simulink library "PTOSim_Lib"  (R2021b)
settings: Solver=ode45  StartTime=0.0  StopTime=10.0  RelTol=1e-3  EnableMultiTasking=on
undefined symbols (not defined in the file or in its folder): DiscIntNeverNeededParam, PTOSimBlock, simu
libraries: $bdroot x3, simulink x2
(part 1 of 2)
settings Model: RequirementInfo="{}  %GIDa_42666abb_d6d9_408c_ae24_f6520282b61c"  Creator=sor  LastModifiedBy=jleonqu
settings SolverCC: AlgebraicLoopSolver=TrustRegion
settings DataIOCC: LimitDataPoints=on  SaveFormat=Array  ReturnWorkspaceOutputs=off
settings OptimizationCC: LifeSpan=inf
settings DebuggingCC: SolverPrmCheckMsg=warning  AllowSymbolicDim=off  SFUnexpectedBacktrackingDiag=warning  SFNoUnconditionalDefaultTransitionDiag=warning  SFExecutionAtInitializationDiag=none  SFMachineParentedDataDiag=warning  ArithmeticOperatorsInVariantConditions=warning
settings HardwareCC: ProdBitPerPointer=32  ProdBitPerSizeT=32  ProdBitPerPtrDiffT=32  ProdLargestAtomicFloat=None  ProdIntDivRoundTo=Undefined  ProdEndianess=Unspecified  ProdWordSize=32  ProdHWDeviceType=32-bit Generic
settings ModelReferenceCC: PropagateSignalLabelsOutOfModel=off
settings SFSimCC: SimUseLocalCustomCode=off  CustomCodeUndefinedFunction=UseInterfaceOnly
settings RTWCC: RTWUseLocalCustomCode=off
settings CodeAppCC: StateflowObjectComments=on
settings GRTTargetCC: TargetLangStandard=C89/C90 (ANSI)
settings ConfigComp: CovMetricSettings=dw  CovSaveCumulativeToWorkspaceVar=on  CovSaveSingleToWorkspaceVar=on  CovExternalEMLEnable=off  CovSFcnEnable=off

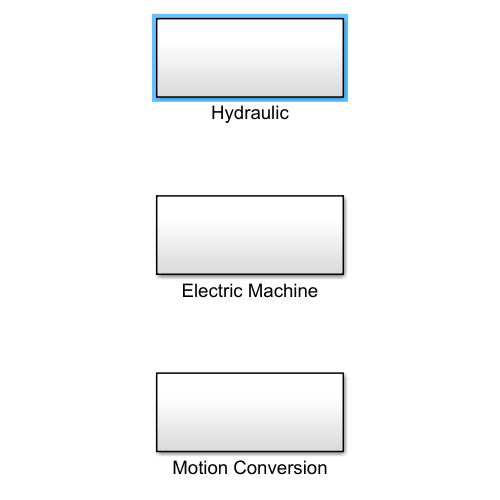
[thumbnail: Simulink's stored preview of the top-level diagram]
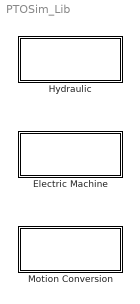
== system PTOSim_Lib ==
  Electric Machine : Subsystem  RequirementInfo="{}  %GIDa_5439fdb4_7c29_433c_8677_23bf92e18f11"
  Hydraulic : Subsystem  RequirementInfo={} %GIDa_f12a42eb_b9cb_4818_b573_b7dee4183a3b
  Motion Conversion : Subsystem

== system PTOSim_Lib/Electric Machine ==
  Electric Generator Equivalent Circuit : Subsystem  mask{PTOSimBlock=PTOSimBlock(1), InputFiletext=Use PTO-Sim input file to define Electric Machine parameters, Ra=0, La=0, Ke=0, bShaft=0, Jem=0}
      mask prompts: PTOSimBlock "Electric Machine Name"; Ra "Armature Resistance [ohm]"; La "Armature Inductance [H]"; Ke "Back-emf or Torque constant [V/(rad/s)]"; bShaft "Rotor Damping [N s/m]"; Jem "Rotor Inertia [kg m^2]"
      mask init:
      | if exist('PTOSimBlock','var')
      |     h=[gcb '/To Workspace'];
      |     responseName=['PTOSimBlock' num2str(PTOSimBlock.PTOSimBlockNum) '_out'];
      |     set_param(h,'VariableName',responseName);
      | end
      | clear h responseName
      | %HydraulicBlock.checkLoc('W');
      settings: PortSchema="{\"entries\":[{\"content\":{\"sides\":[{\"content\":{\"connectorIds\":[\"In1\"]},\"type\":\"ConnectorPlacement.EquallySpacedRectSide\",\"uuid\":\"38b15b7d-d952-45b6-9eb0-5d473736364e\"},{\"content\":{\"connectorIds\":[\"Out1\"],\"side\":\"RIGHT\"},\"type\":\"ConnectorPlacement.EquallySpacedRectSide\",\"uuid\":\"de64adb9-f2de-4dd5-b519-c63af884483d\"},{\"content\":{\"connectorIds\":[\"In2\"],\"side\":\"TOP\"},\"type\":\"ConnectorPlacement.EquallySpacedRectSide\",\"uuid\":\"eaa9506a-5e37-41b4-975c-a8d526700d36\"},{\"content\":{\"connectorIds\":[],\"side\":\"HIDDEN\"},\"type\":\"ConnectorPlacement.EquallySpacedRectSide\",\"uuid\":\"f8da1221-e5bc-4844-b966-beaaa1d6bf60\"}]},\"type\":\"ConnectorPlacement.EquallySpacedConnector\",\"uuid\":\"4da2b473-e94d-42dc-9143-64fbcbf5d9e1\"}],\"packageUris\":[\"http://schema.mathworks.com/mf0/Connector/R2020b\"],\"version\":\"1.0\"}"
      mask DialogControl ParameterGroupVar Prompt: Custom Parameters
      mask DialogControl EMParameters Prompt: Electric Machine Parameters
      mask Display: image('ElectricMotor.png'); % Use "Edit Image" on toolstrip to change.

== system PTOSim_Lib/Hydraulic ==
  Check Valve : Subsystem  mask{PTOSimBlock=PTOSimBlock(1), InputFileText=Use WEC-Sim input file to define Check Valve parameters, pMax=0, pMin=0, Amin=0, Amax=0, rho=0, cd=0, k1=0, k2=0}
      mask prompts: PTOSimBlock "Chack Valve Name"; pMax "Pressure difference at valve maximum opening [Pa]"; pMin "Pressure difference at valve minimum opening [Pa]"; Amin "Minimum valve area [m^2]"; Amax "Maximum valve area [m^2]"; rho "Fluid density [kg/m^3]"; cd "Discharge coefficient"; k1 "Valve coefficient k1 [m^2/N]"; k2 "Valve coefficient k2 [m^2/N]"
      mask init:
      | if exist('PTOSimBlock','var')
      |     h=[gcb '/To Workspace'];
      |     responseName=['PTOSimBlock' num2str(PTOSimBlock.PTOSimBlockNum) '_out'];
      |     set_param(h,'VariableName',responseName);
      | end
      | clear h responseName
      mask DialogControl ParameterGroupVar Prompt: Custom Parameters
      mask DialogControl CheckValveProperties Prompt: Check Valve Properties
      mask Display: image('CheckValve.png'); % Use "Edit Image" on toolstrip to change.
  Compressible Fluid Piston : Subsystem  mask{PTOSimBlock=PTOSimBlock(1), InputFileText=Use WEC-Sim input file to define the Conmpressible Fluid Piston parameters, Ap_A=0, Ap_B=0, PistonStroke=0, BulkModulus=0, xi_piston=0, pAi=0, pBi=0}
      mask prompts: PTOSimBlock "Piston Name"; Ap_A "Piston area A [m]"; Ap_B "Piston area B [m]"; PistonStroke "Piston stroke [m]"; BulkModulus "Fluid Bulk Modulus [Pa]"; xi_piston "Piston initial displacement from A [m]"; pAi "Port A Initial pressure [Pa]"; pBi "Port B Initial pressure [Pa]"
      mask help:
      | PTO-Sim Compressible Fluid Piston
      |
      | This block simualtes a hydraulic cylinder using a compressible fluid model. The block inputs are Response, QA and QB. Response is the signal output of the block Rotational PTO Actuation Force. QA and QB are the flow rate for port A and port B of the cylinder. The outputs of the block are ForcePTO, PA, and PB.
      mask init: same as PTOSim_Lib/Electric Machine/Electric Generator Equivalent Circuit
      settings: PortSchema="{\"entries\":[{\"content\":{\"sides\":[{\"content\":{\"connectorIds\":[\"In1\",\"In2\"]},\"type\":\"ConnectorPlacement.EquallySpacedRectSide\",\"uuid\":\"572dbc7c-8f4c-46fc-9000-663c89355fbd\"},{\"content\":{\"connectorIds\":[\"Out1\",\"Out2\",\"Out3\"],\"side\":\"RIGHT\"},\"type\":\"ConnectorPlacement.EquallySpacedRectSide\",\"uuid\":\"3b7821ce-a540-4de1-8f34-0d55375c774c\"},{\"content\":{\"connectorIds\":[\"In3\"],\"side\":\"TOP\"},\"type\":\"ConnectorPlacement.EquallySpacedRectSide\",\"uuid\":\"b6f5c275-868d-447d-b609-cdda14e9f222\"},{\"content\":{\"connectorIds\":[],\"side\":\"HIDDEN\"},\"type\":\"ConnectorPlacement.EquallySpacedRectSide\",\"uuid\":\"5b34aa5d-01fb-4d75-9f22-3e4ce64ee132\"}]},\"type\":\"ConnectorPlacement.EquallySpacedConnector\",\"uuid\":\"5b16a2f7-6624-4a26-89bf-8d87cef610e1\"}],\"packageUris\":[\"http://schema.mathworks.com/mf0/Connector/R2020b\"],\"version\":\"1.0\"}"
      mask Help:
      | This block simualtes a hydraulic cylinder using a compressible fluid model. The block inputs are Response and HydraulicInput. Response is the signal output of the block Rotational PTO Actuation Force. HydraulicInput is a two signal vector with the information of the flow rate for port A and port B of the cylinder. The output of the block is PistonOutput, which is a three signal vector with PressureA, PressureB, and ForcePTO.
      | 
      | The outputs are calculated using the model presented in the following link: http://wec-sim.github.io/WEC-Sim/master/user/advanced_features.html#pto-sim
      mask DialogControl ParameterGroupVar Prompt: Custom Parameters
      mask DialogControl PistonProperties Prompt: Piston Properties
      mask DialogControl InitialConditions Prompt: Initial Conditions
      mask Display: image('DoubleActingPiston.png'); % Use "Edit Image" on toolstrip to change.
  Gas-Charged Hydraulic Accumulator : Subsystem  mask{PTOSimBlock=PTOSimBlock(1), InputFileText=Use WEC-Sim input file to define Hydraulic Accumulator parameters, VI0=0, VIeq=0, pIprecharge=0}
      mask prompts: PTOSimBlock "Accumulator Name"; VI0 "Total Volume [m^3]"; VIeq "Initial Volume [m^3]"; pIprecharge "Precharge [Pa]"
      mask init: same as PTOSim_Lib/Electric Machine/Electric Generator Equivalent Circuit
      mask DialogControl ParameterGroupVar Prompt: Custom Parameters
      mask DialogControl AccProperties Prompt: Accumulator Properties
      mask Display: image('GasAccumulator.png'); % Use "Edit Image" on toolstrip to change.
  Hydraulic Motor : Subsystem  Variant=on  AllowZeroVariantControls=on  mask{PTOSimBlock=PTOSimBlock(1), InputFileText=Use WEC-Sim input file to define PTO parameters, Displacement=0, effModelVar=Analytical, EffTableDeltaP=0, EffTableShaftSpeed=0, EffTableMechEff=0, EffTableVolEff=0, wNominal=0, deltaPNominal=0, VisNominal=0, DensityNominal=0, EffVolNom=0, TorqueNoLoad=0, TorqueVsPressure=0, rho=0, Viscosity=0}
      mask prompts: PTOSimBlock "Hydraulic Motor Name"; Displacement "Displacement [cc/rev]"; effModelVar "Efficiency Model"; EffTableDeltaP "Pressure data [Pa]"; EffTableShaftSpeed "Shaft speed data [rpm]"; EffTableMechEff "Mechanical Efficiency"; EffTableVolEff "Volumetric Efficiency"; wNominal "Nominal shaft speed [rpm]"; deltaPNominal "Nominal pressure [Pa]"; VisNominal "Nominal viscosity [m^2/s]"; DensityNominal "Nominal density [kg/m^3]"; EffVolNom "Nominal volumetric efficiency"; TorqueNoLoad "No load torque [Nm]"; TorqueVsPressure "Friction torque vs pressure coefficient [Nm/Pa]"; rho "Fluid density [kg/m^3]"; Viscosity "Fluid viscosity [m^2/s]"
      mask init:
      | if exist('PTOSimBlock','var')
      |     %%
      |     % Analytical efficiency
      |     %%
      |     h = [gcb '/AnalyticalEfficiencyModel'];
      |     responseName = ['sv_b' num2str(PTOSimBlock.PTOSimBlockNum) '_AnalyticalEfficiency'];
      |     set_param(h,'VariantControl',responseName);
      |     %%
      |     % Tabulated Efficiency
      |     %%
      |     h = [gcb '/TabulatedEfficiency'];
      |     responseName = ['sv_b' num2str(PTOSimBlock.PTOSimBlockNum) '_TabulatedEfficiency'];
      |     set_param(h,'VariantControl',responseName);
      |     %%
      |     % Set zero active variant controls to prevent label issue (works 2017b+)
      |     %%
      |     set_param(gcb,'AllowZeroVariantControls','on');
      |     %%
      |     h=[gcb '/TabulatedEfficiency/To Workspace'];
      |     responseName=['PTOSimBlock' num2str(PTOSimBlock.PTOSimBlockNum) '_out'];
      |     set_param(h,'VariableName',responseName);
      |     %%
      |     h=[gcb '/AnalyticalEfficiencyModel/To Workspace'];
      |     responseName=['PTOSimBlock' num2str(PTOSimBlock.PTOSimBlockNum) '_out'];
      |     set_param(h,'VariableName',responseName);
      | end
      | clear h responseName
      mask TypeOptions effModelVar: Analytical | Tabulated
      mask Callback effModelVar: ptoSimClassCallback(gcbh)
      mask DialogControl ParameterGroupVar Prompt: Custom Parameters
      mask DialogControl HMProperties Prompt: Hydraulic Motor Properties
      mask Display: image('VariableDisplacementHydraulicMotor.png'); % Use "Edit Image" on toolstrip to change.
  Rectifying Check Valve : Subsystem  mask{PTOSimBlock=PTOSimBlock(1), InputFileText=Use PTO-Sim input file to define PTO parameters, Cd=0, Amax=0, Amin=0, pMin=0, pMax=0, rho=0, k1=0, k2=0}
      mask prompts: PTOSimBlock "Rectifying Valve Name"; Cd "Discharge coefficient"; Amax "Maximum opening area"; Amin "Minimum opening Area"; pMin "Cracking pressure"; pMax "Pressure at maximum opening"; rho "Fluid density"; k1 "Valve Coefficient k1"; k2 "Valve Coefficient k2"
      mask init: same as PTOSim_Lib/Electric Machine/Electric Generator Equivalent Circuit
      mask DialogControl ParameterGroupVar Prompt: Custom Parameters
      mask DialogControl CheckValveProperties Prompt: Check valve properties
      mask Display: image('RectifyingCheckValve.png'); % Use "Edit Image" on toolstrip to change.

== system PTOSim_Lib/Motion Conversion ==
  Rotary to Linear Adjustable Rod : Subsystem  mask{PTOSimBlock=PTOSimBlock(1), InputFiletext=Use WEC-Sim input file to define Adjustable Rod parameters, crank=0, offset=0, rodInit=0}
      mask prompts: PTOSimBlock "Adjustable Rod Name"; crank "Crank [m]"; offset "Offset [m]"; rodInit "Rod initial position [m]"
      mask init: same as PTOSim_Lib/Hydraulic/Check Valve
      mask DialogControl ParameterGroupVar Prompt: Custom Parameters
      mask DialogControl AdjRodParameters Prompt: Adjustable Rod Properties
  Rotary to Linear Crank : Subsystem  mask{PTOSimBlock=PTOSimBlock(1), InputFiletext=Use WEC-Sim input file to define Linear Crank parameters, crank=0, offset=0, rodLength=0}
      mask prompts: PTOSimBlock "Linear Crank Name"; crank "Crank [m]"; offset "Offset [m]"; rodLength "Rod length [m]"
      mask init: same as PTOSim_Lib/Hydraulic/Check Valve
      mask DialogControl ParameterGroupVar Prompt: Custom Parameters
      mask DialogControl LinCrankParameters Prompt: Linear Crank Parameters

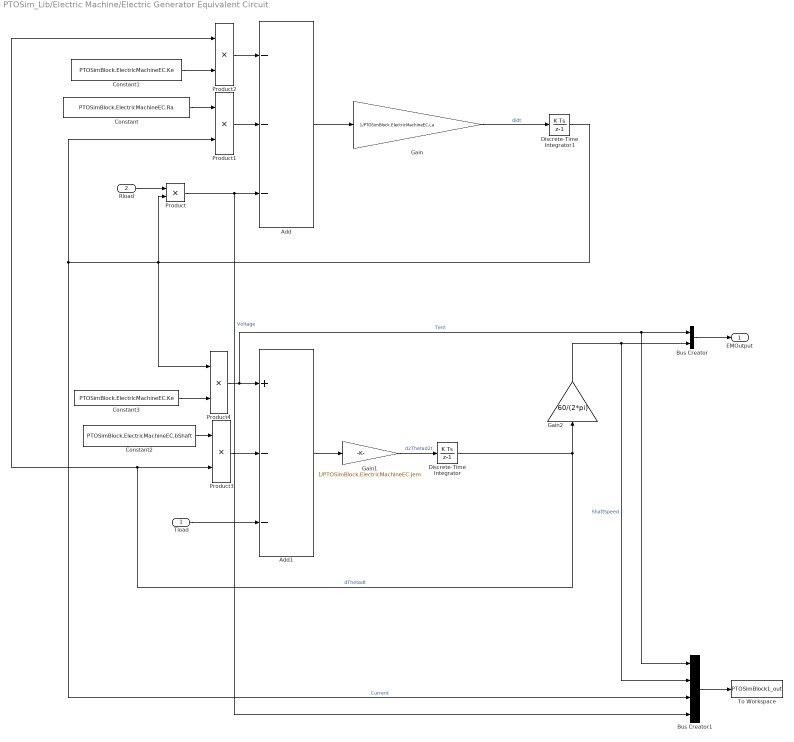
== system PTOSim_Lib/Electric Machine/Electric Generator Equivalent Circuit ==
  Tload : Inport
  Rload : Inport  Port=2
  Add : Sum  Inputs=---
  Add1 : Sum  Inputs=+--
  Bus Creator : BusCreator  Inputs=2
  Bus Creator1 : BusCreator  Inputs=4
  Constant : Constant  Value=PTOSimBlock.ElectricMachineEC.Ra
  Constant1 : Constant  Value=PTOSimBlock.ElectricMachineEC.Ke
  Constant2 : Constant  Value=PTOSimBlock.ElectricMachineEC.bShaft
  Constant3 : Constant  Value=PTOSimBlock.ElectricMachineEC.Ke
  Discrete-Time Integrator : DiscreteIntegrator  SampleTime=-1  ICPrevOutput=DiscIntNeverNeededParam  ICPrevScaledInput=DiscIntNeverNeededParam
  Discrete-Time Integrator1 : DiscreteIntegrator  SampleTime=-1  ICPrevOutput=DiscIntNeverNeededParam  ICPrevScaledInput=DiscIntNeverNeededParam
  Gain : Gain  Gain=1/PTOSimBlock.ElectricMachineEC.La
  Gain1 : Gain  Gain=1/PTOSimBlock.ElectricMachineEC.Jem
  Gain2 : Gain  Gain=60/(2*pi)
  Product{,1..4} (5 alike) : Product
  To Workspace : ToWorkspace  VariableName=PTOSimBlock1_out  SaveFormat=Structure With Time  SampleTime=simu.dtOut
  EMOutput : Outport
  wires:
  Add/1 -> Gain/1
  Gain/1 -> Discrete-Time Integrator1/1  "didt"
  Rload/1 -> Product/1
  Discrete-Time Integrator1/1 -> Product4/1, Product/2, Bus Creator1/3, Product1/2  "Current"
  Product/1 -> Bus Creator1/4, Add/3  "Voltage"
  Product1/1 -> Add/2
  Constant/1 -> Product1/1
  Product2/1 -> Add/1
  Constant1/1 -> Product2/2
  Tload/1 -> Add1/3
  Add1/1 -> Gain1/1
  Gain1/1 -> Discrete-Time Integrator/1  "d2Thetad2t"
  Product3/1 -> Add1/2
  Constant2/1 -> Product3/1
  Discrete-Time Integrator/1 -> Product2/1, Product3/2, Gain2/1  "dThetadt"
  Product4/1 -> Bus Creator1/1, Bus Creator/1, Add1/1  "Tem"
  Constant3/1 -> Product4/2
  Bus Creator/1 -> EMOutput/1
  Gain2/1 -> Bus Creator1/2, Bus Creator/2  "ShaftSpeed"
  Bus Creator1/1 -> To Workspace/1

== system PTOSim_Lib/Hydraulic/Check Valve ==
  DeltaP : Inport
  Bus Creator : BusCreator  Inputs=2
  Constant : Constant  Value=PTOSimBlock.CheckValve.rho
  Divide : Product  Inputs=/*
  Gain : Gain  Gain=PTOSimBlock.CheckValve.k1
  Gain1 : Gain  Gain=2
  Gain2 : Gain  Gain=PTOSimBlock.CheckValve.Cd
  Product : Product
  Product1 : Product
  Sqrt : Sqrt  SaturateOnIntegerOverflow=on
  Subsystem : Subsystem
  To Workspace : ToWorkspace  VariableName=PTOSimBlock1_out  SaveFormat=Structure With Time  SampleTime=-1
  Trigonometric Function : Trigonometry  Operator=tanh
  Qcv : Outport
  wires:
  Product1/1 -> Bus Creator/1, Qcv/1  "FlowCheckValve"
  DeltaP/1 -> Bus Creator/2, Subsystem/1(DeltaP), Gain/1, Gain1/1  "DeltaPCheckValve"
  Subsystem/1(Av) -> Product1/2
  Gain/1 -> Trigonometric Function/1
  Trigonometric Function/1 -> Product/1
  Gain1/1 -> Product/2
  Sqrt/1 -> Gain2/1
  Divide/1 -> Sqrt/1
  Gain2/1 -> Product1/1
  Constant/1 -> Divide/1
  Product/1 -> Divide/2
  Bus Creator/1 -> To Workspace/1

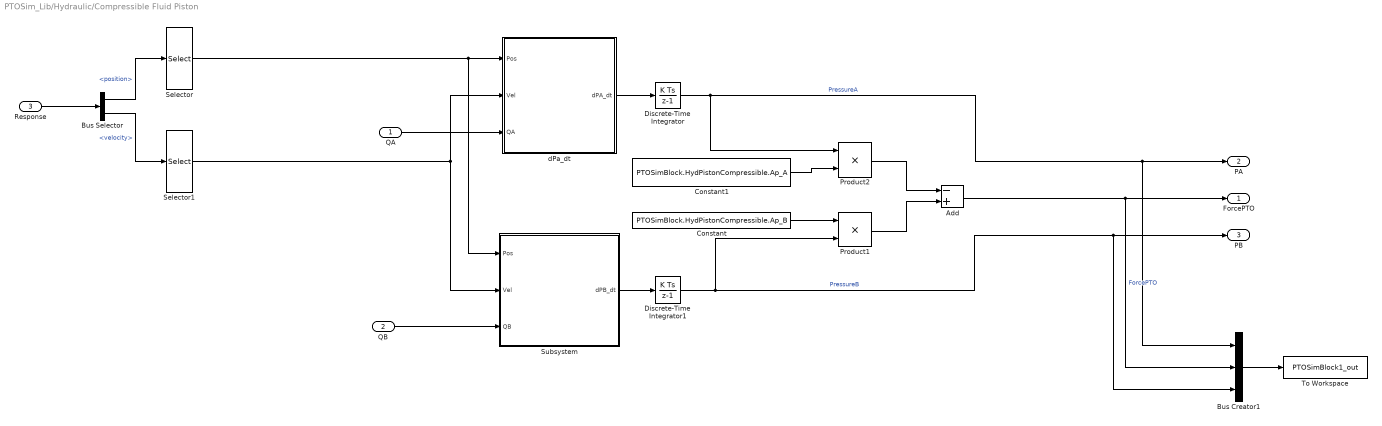
== system PTOSim_Lib/Hydraulic/Compressible Fluid Piston ==
  QA : Inport
  QB : Inport  Port=2
  Response : Inport  Port=3
  Add : Sum  Inputs=-+
  Bus Creator1 : BusCreator  Inputs=3
  Bus Selector : BusSelector  OutputSignals=position,velocity
  Constant : Constant  Value=PTOSimBlock.HydPistonCompressible.Ap_B
  Constant1 : Constant  Value=PTOSimBlock.HydPistonCompressible.Ap_A
  Discrete-Time Integrator : DiscreteIntegrator  InitialCondition=PTOSimBlock.HydPistonCompressible.pAi  SampleTime=-1  ICPrevOutput=DiscIntNeverNeededParam  ICPrevScaledInput=DiscIntNeverNeededParam
  Discrete-Time Integrator1 : DiscreteIntegrator  InitialCondition=PTOSimBlock.HydPistonCompressible.pBi  SampleTime=-1  ICPrevOutput=DiscIntNeverNeededParam  ICPrevScaledInput=DiscIntNeverNeededParam
  Product1 : Product
  Product2 : Product
  Selector : Selector  InputPortWidth=6  IndexOptions=Index vector (dialog)  Indices=3  OutputSizes=1
  Selector1 : Selector  InputPortWidth=6  IndexOptions=Index vector (dialog)  Indices=3  OutputSizes=1
  Subsystem : Subsystem  AncestorBlock=PTOSim_Lib_UpdatedV3/Hydraulic/Compressible Fluid Piston Updated/Subsystem
  To Workspace : ToWorkspace  VariableName=PTOSimBlock1_out  SaveFormat=Structure With Time  SampleTime=simu.dtOut
  dPa_dt : Subsystem  AncestorBlock=PTOSim_Lib_UpdatedV3/Hydraulic/Compressible Fluid Piston Updated/dPa_dt
  ForcePTO : Outport
  PA : Outport  Port=2
  PB : Outport  Port=3
  wires:
  QA/1 -> dPa_dt/3(QA)
  Constant1/1 -> Product2/2
  Discrete-Time Integrator1/1 -> Bus Creator1/3, PB/1, Product1/2  "PressureB"
  Selector/1 -> Subsystem/1(Pos), dPa_dt/1(Pos)
  Add/1 -> Bus Creator1/2, ForcePTO/1  "ForcePTO"
  Bus Creator1/1 -> To Workspace/1
  QB/1 -> Subsystem/3(QB)
  Product1/1 -> Add/2
  dPa_dt/1(dPA_dt) -> Discrete-Time Integrator/1
  Product2/1 -> Add/1
  Constant/1 -> Product1/1
  Bus Selector/2 -> Selector1/1  "<velocity>"
  Subsystem/1(dPB_dt) -> Discrete-Time Integrator1/1
  Selector1/1 -> Subsystem/2(Vel), dPa_dt/2(Vel)
  Response/1 -> Bus Selector/1
  Discrete-Time Integrator/1 -> PA/1, Bus Creator1/1, Product2/1  "PressureA"
  Bus Selector/1 -> Selector/1  "<position>"

== system PTOSim_Lib/Hydraulic/Gas-Charged Hydraulic Accumulator ==
  FlowRate : Inport
  Add1 : Sum  Inputs=-+
  Bus Creator : BusCreator  Inputs=2
  Constant4 : Constant  Value=PTOSimBlock.GasHydAccumulator.pIprecharge
  Constant5 : Constant  Value=PTOSimBlock.GasHydAccumulator.VI0
  Constant6 : Constant  Value=PTOSimBlock.GasHydAccumulator.VI0
  Constant7 : Constant  Value=1.4
  Discrete-Time Integrator1 : DiscreteIntegrator  SampleTime=-1  ICPrevOutput=DiscIntNeverNeededParam  ICPrevScaledInput=DiscIntNeverNeededParam
  Divide2 : Product  Inputs=*/
  Math Function1 : Math  Operator=pow  SaturateOnIntegerOverflow=on
  Product : Product
  To Workspace : ToWorkspace  VariableName=PTOSimBlock1_out  SaveFormat=Structure With Time  SampleTime=simu.dtOut
  Pressure : Outport
  wires:
  Constant4/1 -> Product/1
  Constant5/1 -> Divide2/1
  Constant6/1 -> Add1/2
  Discrete-Time Integrator1/1 -> Add1/1
  FlowRate/1 -> Bus Creator/2, Discrete-Time Integrator1/1  "FlowRate"
  Add1/1 -> Divide2/2
  Divide2/1 -> Math Function1/1
  Constant7/1 -> Math Function1/2
  Math Function1/1 -> Product/2
  Product/1 -> Bus Creator/1, Pressure/1  "Pressure"
  Bus Creator/1 -> To Workspace/1

== system PTOSim_Lib/Hydraulic/Hydraulic Motor ==
  note: 1) Add Subsystem or Model blocks as valid variant choices.
      | 2) You cannot connect blocks at this level. At simulation, connectivity is automatically
      | determined, based on the active variant and port name matching.
  Displ : Inport
  DeltaP : Inport  Port=2
  ShaftSpeed : Inport  Port=3
  AnalyticalEfficiencyModel : Subsystem  VariantControl=sv_b1_AnalyticalEfficiency
  TabulatedEfficiency : Subsystem  VariantControl=sv_b1_TabulatedEfficiency
  Torque : Outport
  FlowRate : Outport  Port=2

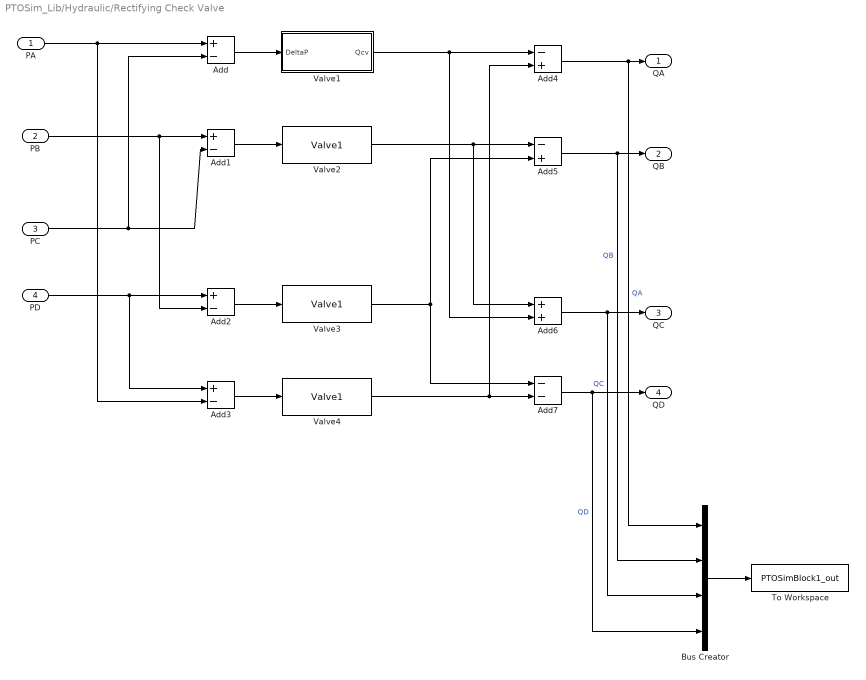
== system PTOSim_Lib/Hydraulic/Rectifying Check Valve ==
  PA : Inport
  PB : Inport  Port=2
  PC : Inport  Port=3
  PD : Inport  Port=4
  Add{,1..3} (4 alike) : Sum  Inputs=+-
  Add4 : Sum  Inputs=-+
  Add5 : Sum  Inputs=-+
  Add6 : Sum
  Add7 : Sum  Inputs=--
  Bus Creator : BusCreator  Inputs=4
  To Workspace : ToWorkspace  VariableName=PTOSimBlock1_out  SaveFormat=Structure With Time  SampleTime=-1
  Valve1 : Subsystem
  Valve2 : $bdroot/Hydraulic/Rectifying Check Valve/Valve1  SystemSampleTime=-1  VariantActivationTime=update diagram  Latency=0  AutoFrameSizeCalculation=off
  Valve3 : $bdroot/Hydraulic/Rectifying Check Valve/Valve1  SystemSampleTime=-1  VariantActivationTime=update diagram  Latency=0  AutoFrameSizeCalculation=off
  Valve4 : $bdroot/Hydraulic/Rectifying Check Valve/Valve1  SystemSampleTime=-1  VariantActivationTime=update diagram  Latency=0  AutoFrameSizeCalculation=off
  QA : Outport
  QB : Outport  Port=2
  QC : Outport  Port=3
  QD : Outport  Port=4
  wires:
  Add/1 -> Valve1/1(DeltaP)
  PA/1 -> Add3/2, Add/1
  PC/1 -> Add/2, Add1/2
  Add1/1 -> Valve2/1
  PB/1 -> Add2/2, Add1/1
  Add2/1 -> Valve3/1
  PD/1 -> Add3/1, Add2/1
  Add3/1 -> Valve4/1
  Valve1/1(Qcv) -> Add6/2, Add4/1
  Valve4/1 -> Add7/2, Add4/2
  Valve2/1 -> Add6/1, Add5/1
  Valve3/1 -> Add7/1, Add5/2
  Add7/1 -> Bus Creator/4, QD/1  "QD"
  Add6/1 -> Bus Creator/3, QC/1  "QC"
  Add5/1 -> Bus Creator/2, QB/1  "QB"
  Bus Creator/1 -> To Workspace/1
  Add4/1 -> Bus Creator/1, QA/1  "QA"

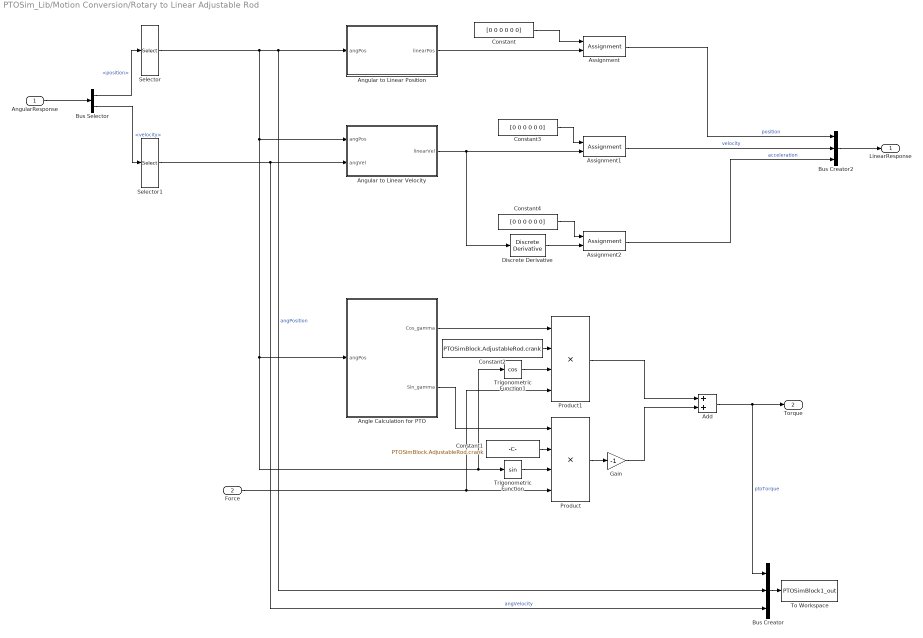
== system PTOSim_Lib/Motion Conversion/Rotary to Linear Adjustable Rod ==
  AngularResponse : Inport
  Force : Inport  Port=2
  Add : Sum
  Angle Calculation for PTO : Subsystem
  Angular to Linear Position : Subsystem
  Angular to Linear Velocity : Subsystem
  Assignment : Assignment  IndexOptions=Index vector (dialog)  Indices=3  OutputSizes=1
  Assignment1 : Assignment  IndexOptions=Index vector (dialog)  Indices=3  OutputSizes=1
  Assignment2 : Assignment  IndexOptions=Index vector (dialog)  Indices=3  OutputSizes=1
  Bus Creator : BusCreator  Inputs=3
  Bus Creator2 : BusCreator  Inputs=3
  Bus Selector : BusSelector  OutputSignals=position,velocity
  Constant : Constant  Value=[0 0 0 0 0 0]
  Constant1 : Constant  Value=PTOSimBlock.AdjustableRod.crank
  Constant2 : Constant  Value=PTOSimBlock.AdjustableRod.crank
  Constant3 : Constant  Value=[0 0 0 0 0 0]
  Constant4 : Constant  Value=[0 0 0 0 0 0]
  Discrete Derivative : simulink/Discrete/Discrete Derivative  gainval=1.0  ICPrevScaledInput=0.0  OutMin=[]  OutMax=[]  OutDataType=fixdt(1, 16)  OutScaling=2^-10  DoSatur=off
  Gain : Gain  Gain=-1
  Product : Product  Inputs=4
  Product1 : Product  Inputs=4
  Selector : Selector  InputPortWidth=6  IndexOptions=Index vector (dialog)  Indices=5  OutputSizes=1
  Selector1 : Selector  InputPortWidth=6  IndexOptions=Index vector (dialog)  Indices=5  OutputSizes=1
  To Workspace : ToWorkspace  VariableName=PTOSimBlock1_out  SaveFormat=Structure With Time  SampleTime=-1
      settings: Decimation=round(simu.dtOut/simu.dt,0)
  Trigonometric Function : Trigonometry
  Trigonometric Function1 : Trigonometry  Operator=cos
  LinearResponse : Outport
  Torque : Outport  Port=2
  wires:
  Angular to Linear Position/1(linearPos) -> Assignment/2
  Selector1/1 -> Bus Creator/3, Angular to Linear Velocity/2(angVel)  "angVelocity"
  Add/1 -> Torque/1, Bus Creator/1  "ptoTorque"
  Bus Creator/1 -> To Workspace/1
  Selector/1 -> Angular to Linear Velocity/1(angPos), Trigonometric Function1/1, Trigonometric Function/1, Angle Calculation for PTO/1(angPos), Bus Creator/2, Angular to Linear Position/1(angPos)  "angPosition"
  Product1/1 -> Add/1
  Gain/1 -> Add/2
  Angle Calculation for PTO/2(Sin_gamma) -> Product/1
  Trigonometric Function1/1 -> Product1/3
  Angle Calculation for PTO/1(Cos_gamma) -> Product1/1
  Force/1 -> Product1/4, Product/4
  Constant2/1 -> Product1/2
  Trigonometric Function/1 -> Product/3
  Constant1/1 -> Product/2
  Product/1 -> Gain/1
  Constant/1 -> Assignment/1
  Constant3/1 -> Assignment1/1
  Angular to Linear Velocity/1(linearVel) -> Discrete Derivative/1, Assignment1/2
  Assignment/1 -> Bus Creator2/1  "position"
  Assignment1/1 -> Bus Creator2/2  "velocity"
  Constant4/1 -> Assignment2/1
  Discrete Derivative/1 -> Assignment2/2
  Assignment2/1 -> Bus Creator2/3  "acceleration"
  Bus Creator2/1 -> LinearResponse/1
  Bus Selector/1 -> Selector/1  "<position>"
  Bus Selector/2 -> Selector1/1  "<velocity>"
  AngularResponse/1 -> Bus Selector/1

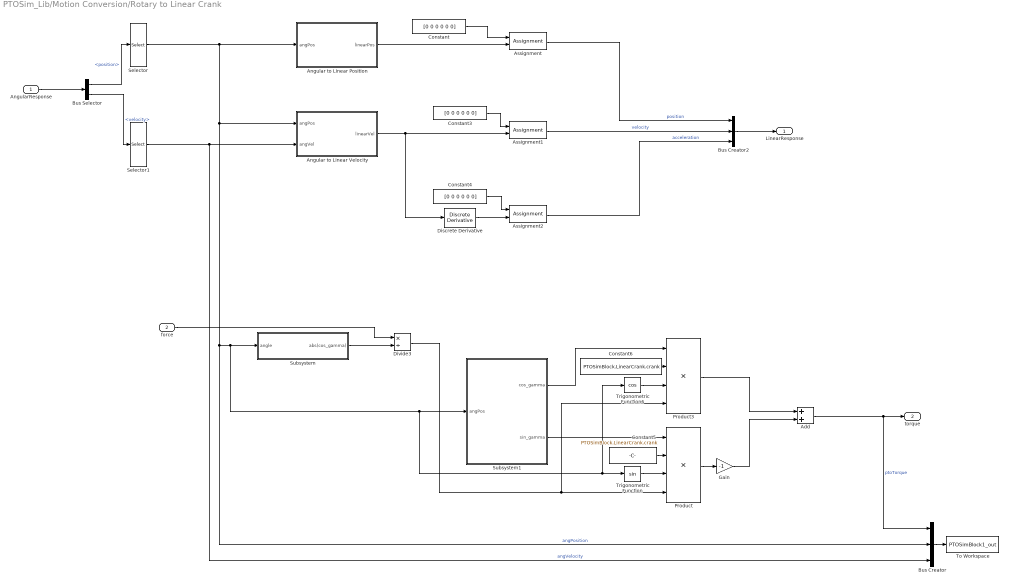
== system PTOSim_Lib/Motion Conversion/Rotary to Linear Crank ==
  AngularResponse : Inport
  force : Inport  Port=2
  Add : Sum
  Angular to Linear Position : Subsystem
  Angular to Linear Velocity : Subsystem
  Assignment : Assignment  IndexOptions=Index vector (dialog)  Indices=3  OutputSizes=1
  Assignment1 : Assignment  IndexOptions=Index vector (dialog)  Indices=3  OutputSizes=1
  Assignment2 : Assignment  IndexOptions=Index vector (dialog)  Indices=3  OutputSizes=1
  Bus Creator : BusCreator  Inputs=3
  Bus Creator2 : BusCreator  Inputs=3
  Bus Selector : BusSelector  OutputSignals=position,velocity
  Constant : Constant  Value=[0 0 0 0 0 0]
  Constant3 : Constant  Value=[0 0 0 0 0 0]
  Constant4 : Constant  Value=[0 0 0 0 0 0]
  Constant5 : Constant  Value=PTOSimBlock.LinearCrank.crank
  Constant6 : Constant  Value=PTOSimBlock.LinearCrank.crank
  Discrete Derivative : simulink/Discrete/Discrete Derivative  gainval=1.0  ICPrevScaledInput=0.0  OutMin=[]  OutMax=[]  OutDataType=fixdt(1, 16)  OutScaling=2^-10  DoSatur=off
  Divide3 : Product  Inputs=*/
  Gain : Gain  Gain=-1
  Product : Product  Inputs=4
  Product3 : Product  Inputs=4
  Selector : Selector  InputPortWidth=6  IndexOptions=Index vector (dialog)  Indices=5  OutputSizes=1
  Selector1 : Selector  InputPortWidth=6  IndexOptions=Index vector (dialog)  Indices=5  OutputSizes=1
  Subsystem : Subsystem
  Subsystem1 : Subsystem  AncestorBlock=PTOSim_Lib/Motion Conversion/Rotary to Linear Adjustable Rod/Subsystem
  To Workspace : ToWorkspace  VariableName=PTOSimBlock1_out  SaveFormat=Structure With Time  SampleTime=-1
      settings: Decimation=round(simu.dtOut/simu.dt,0)
  Trigonometric Function : Trigonometry
  Trigonometric Function6 : Trigonometry  Operator=cos
  LinearResponse : Outport
  torque : Outport  Port=2
  wires:
  Selector1/1 -> Bus Creator/3, Angular to Linear Velocity/2(angVel)  "angVelocity"
  Add/1 -> Bus Creator/1, torque/1  "ptoTorque"
  Bus Creator/1 -> To Workspace/1
  Subsystem/1(abs(cos_gamma)) -> Divide3/2
  force/1 -> Divide3/1
  Trigonometric Function6/1 -> Product3/3
  Subsystem1/1(cos_gamma) -> Product3/1
  Constant6/1 -> Product3/2
  Divide3/1 -> Product/4, Product3/4
  Gain/1 -> Add/2
  Product3/1 -> Add/1
  Subsystem1/2(sin_gamma) -> Product/1
  Selector/1 -> Angular to Linear Velocity/1(angPos), Subsystem1/1(angPos), Trigonometric Function/1, Trigonometric Function6/1, Subsystem/1(angle), Bus Creator/2, Angular to Linear Position/1(angPos)  "angPosition"
  Trigonometric Function/1 -> Product/3
  Constant5/1 -> Product/2
  Product/1 -> Gain/1
  Bus Selector/2 -> Selector1/1  "<velocity>"
  Bus Selector/1 -> Selector/1  "<position>"
  AngularResponse/1 -> Bus Selector/1
  Constant/1 -> Assignment/1
  Assignment1/1 -> Bus Creator2/2  "velocity"
  Constant4/1 -> Assignment2/1
  Discrete Derivative/1 -> Assignment2/2
  Angular to Linear Velocity/1(linearVel) -> Discrete Derivative/1, Assignment1/2
  Assignment2/1 -> Bus Creator2/3  "acceleration"
  Constant3/1 -> Assignment1/1
  Assignment/1 -> Bus Creator2/1  "position"
  Angular to Linear Position/1(linearPos) -> Assignment/2
  Bus Creator2/1 -> LinearResponse/1

== system PTOSim_Lib/Hydraulic/Check Valve/Subsystem ==
  DeltaP : Inport
  Add : Sum
  Add1 : Sum  Inputs=+-
  Add2 : Sum  Inputs=+-
  Add3 : Sum
  Add4 : Sum
  Constant : Constant
  Constant1 : Constant  Value=PTOSimBlock.CheckValve.Amax
  Constant2 : Constant  Value=PTOSimBlock.CheckValve.Amin
  Constant3 : Constant  Value=PTOSimBlock.CheckValve.pMax
  Constant4 : Constant  Value=PTOSimBlock.CheckValve.pMin
  Constant5 : Constant  Value=PTOSimBlock.CheckValve.Amin
  Gain : Gain  Gain=PTOSimBlock.CheckValve.k2
  Gain1 : Gain  Gain=0.5
  Gain2 : Gain  Gain=0.5
  Product : Product
  Trigonometric Function : Trigonometry  Operator=tanh
  Av : Outport
  wires:
  Gain1/1 -> Add2/2
  Add2/1 -> Gain/1
  Constant3/1 -> Add3/1
  Constant4/1 -> Add3/2
  Constant2/1 -> Add1/2
  Product/1 -> Add4/2
  Constant5/1 -> Add4/1
  Gain/1 -> Trigonometric Function/1
  DeltaP/1 -> Add2/1
  Constant/1 -> Add/2
  Add1/1 -> Gain2/1
  Gain2/1 -> Product/2
  Trigonometric Function/1 -> Add/1
  Add3/1 -> Gain1/1
  Add/1 -> Product/1
  Constant1/1 -> Add1/1
  Add4/1 -> Av/1

== system PTOSim_Lib/Hydraulic/Compressible Fluid Piston/Subsystem ==
  Pos : Inport
  Vel : Inport  Port=2
  QB : Inport  Port=3
  Add : Sum  Inputs=-+
  Add1 : Sum  Inputs=+-+
  Constant : Constant  Value=PTOSimBlock.HydPistonCompressible.Ap_B
  Constant1 : Constant  Value=PTOSimBlock.HydPistonCompressible.PistonStroke
  Constant2 : Constant  Value=PTOSimBlock.HydPistonCompressible.Ap_B
  Constant3 : Constant  Value=PTOSimBlock.HydPistonCompressible.BulkModulus
  Constant4 : Constant  Value=PTOSimBlock.HydPistonCompressible.xi_piston
  Divide : Product  Inputs=/*
  Product : Product
  Product1 : Product
  Product2 : Product
  Saturation : Saturate  UpperLimit=inf  LowerLimit=1e-10
  dPB_dt : Outport
  wires:
  Saturation/1 -> Divide/1
  Vel/1 -> Product/1
  Constant/1 -> Product/2
  Product/1 -> Add/1
  QB/1 -> Add/2
  Add/1 -> Product1/2
  Pos/1 -> Add1/1
  Add1/1 -> Product2/1
  Constant2/1 -> Product2/2
  Product2/1 -> Saturation/1
  Constant3/1 -> Divide/2
  Divide/1 -> Product1/1
  Product1/1 -> dPB_dt/1
  Constant1/1 -> Add1/3
  Constant4/1 -> Add1/2

== system PTOSim_Lib/Hydraulic/Compressible Fluid Piston/dPa_dt ==
  Pos : Inport
  Vel : Inport  Port=2
  QA : Inport  Port=3
  Add : Sum
  Add1 : Sum  Inputs=+-
  Constant : Constant  Value=PTOSimBlock.HydPistonCompressible.Ap_A
  Constant1 : Constant  Value=PTOSimBlock.HydPistonCompressible.BulkModulus
  Constant2 : Constant  Value=PTOSimBlock.HydPistonCompressible.xi_piston
  Constant3 : Constant  Value=PTOSimBlock.HydPistonCompressible.Ap_A
  Divide : Product  Inputs=/*
  Divide1 : Product  Inputs=*/
  Product : Product
  Product1 : Product
  Saturation : Saturate  UpperLimit=inf  LowerLimit=1e-10
  dPA_dt : Outport
  wires:
  Divide1/1 -> Product1/1
  Constant3/1 -> Divide1/2
  Constant1/1 -> Divide1/1
  Saturation/1 -> Divide/1
  Vel/1 -> Product/1
  Product1/1 -> Divide/2
  Divide/1 -> dPA_dt/1
  Add/1 -> Product1/2
  Constant/1 -> Product/2
  QA/1 -> Add/2
  Product/1 -> Add/1
  Pos/1 -> Add1/2
  Constant2/1 -> Add1/1
  Add1/1 -> Saturation/1

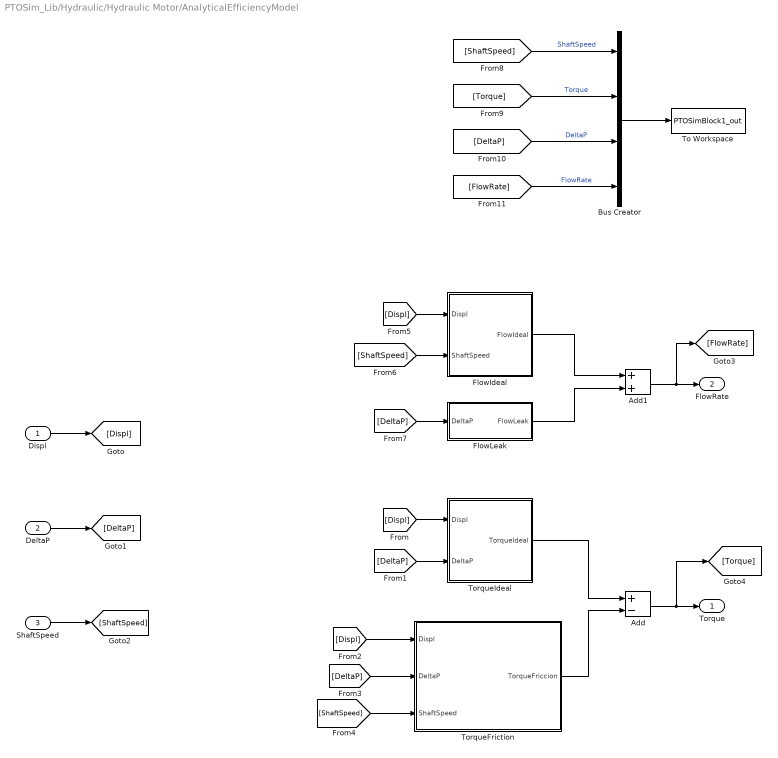
== system PTOSim_Lib/Hydraulic/Hydraulic Motor/AnalyticalEfficiencyModel ==
  Displ : Inport
  DeltaP : Inport  Port=2
  ShaftSpeed : Inport  Port=3
  Add : Sum  Inputs=+-
  Add1 : Sum
  Bus Creator : BusCreator  Inputs=4
  FlowIdeal : Subsystem
  FlowLeak : Subsystem
  To Workspace : ToWorkspace  VariableName=PTOSimBlock1_out  SaveFormat=Structure With Time  SampleTime=-1
  TorqueFriction : Subsystem
  TorqueIdeal : Subsystem
  Torque : Outport
  FlowRate : Outport  Port=2
  wires:
  Bus Creator/1 -> To Workspace/1
  Add/1 -> [Torque], Torque/1
  TorqueIdeal/1(TorqueIdeal) -> Add/1
  TorqueFriction/1(TorqueFriccion) -> Add/2
  Displ/1 -> [Displ]
  DeltaP/1 -> [DeltaP]
  ShaftSpeed/1 -> [ShaftSpeed]
  [Displ] -> TorqueIdeal/1(Displ)
  [DeltaP] -> TorqueIdeal/2(DeltaP)
  [DeltaP] -> TorqueFriction/2(DeltaP)
  [Displ] -> TorqueFriction/1(Displ)
  [ShaftSpeed] -> TorqueFriction/3(ShaftSpeed)
  FlowIdeal/1(FlowIdeal) -> Add1/1
  FlowLeak/1(FlowLeak) -> Add1/2
  Add1/1 -> [FlowRate], FlowRate/1
  [Displ] -> FlowIdeal/1(Displ)
  [ShaftSpeed] -> FlowIdeal/2(ShaftSpeed)
  [DeltaP] -> FlowLeak/1(DeltaP)
  [ShaftSpeed] -> Bus Creator/1  "ShaftSpeed"
  [Torque] -> Bus Creator/2  "Torque"
  [DeltaP] -> Bus Creator/3  "DeltaP"
  [FlowRate] -> Bus Creator/4  "FlowRate"

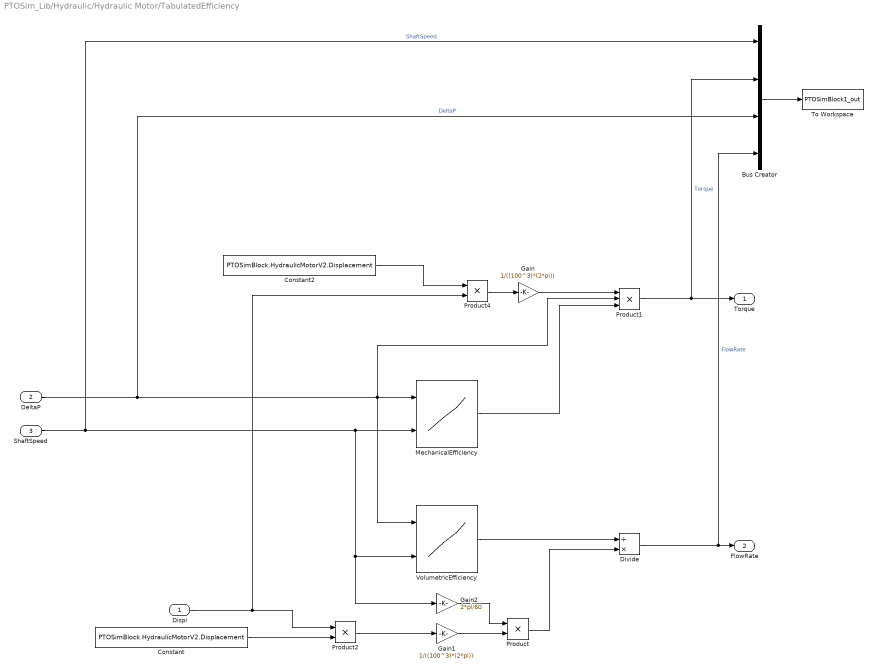
== system PTOSim_Lib/Hydraulic/Hydraulic Motor/TabulatedEfficiency ==
  Displ : Inport
  DeltaP : Inport  Port=2
  ShaftSpeed : Inport  Port=3
  Bus Creator : BusCreator  Inputs=4
  Constant : Constant  Value=PTOSimBlock.HydraulicMotorV2.Displacement
  Constant2 : Constant  Value=PTOSimBlock.HydraulicMotorV2.Displacement
  Divide : Product  Inputs=/*
  Gain : Gain  Gain=1/((100^3)*(2*pi))
  Gain1 : Gain  Gain=1/((100^3)*(2*pi))
  Gain2 : Gain  Gain=2*pi/60
  MechanicalEfficiency : Lookup_n-D  BreakpointsForDimension1=PTOSimBlock.HydraulicMotorV2.EffTableShaftSpeed  BreakpointsForDimension2=PTOSimBlock.HydraulicMotorV2.EffTableDeltaP  Table=PTOSimBlock.HydraulicMotorV2.EffTableMechEff  InternalRulePriority=Speed  RndMeth=Simplest  InputSameDT=on
      settings: InputPortMap=u0,u1
  Product : Product
  Product1 : Product  Inputs=3
  Product2 : Product
  Product4 : Product
  To Workspace : ToWorkspace  VariableName=PTOSimBlock1_out  SaveFormat=Structure With Time  SampleTime=-1
  VolumetricEfficiency : Lookup_n-D  BreakpointsForDimension1=PTOSimBlock.HydraulicMotorV2.EffTableShaftSpeed  BreakpointsForDimension2=PTOSimBlock.HydraulicMotorV2.EffTableDeltaP  Table=PTOSimBlock.HydraulicMotorV2.EffTableVolEff  InternalRulePriority=Speed  RndMeth=Simplest  InputSameDT=on
      settings: InputPortMap=u0,u1
  Torque : Outport
  FlowRate : Outport  Port=2
  wires:
  ShaftSpeed/1 -> MechanicalEfficiency/2, Gain2/1, VolumetricEfficiency/2, Bus Creator/1  "ShaftSpeed"
  Divide/1 -> Bus Creator/4, FlowRate/1  "FlowRate"
  Product1/1 -> Bus Creator/2, Torque/1  "Torque"
  Gain1/1 -> Product/2
  Product/1 -> Divide/2
  Gain/1 -> Product1/1
  VolumetricEfficiency/1 -> Divide/1
  DeltaP/1 -> Product1/2, VolumetricEfficiency/1, MechanicalEfficiency/1, Bus Creator/3  "DeltaP"
  MechanicalEfficiency/1 -> Product1/3
  Product2/1 -> Gain1/1
  Bus Creator/1 -> To Workspace/1
  Product4/1 -> Gain/1
  Constant/1 -> Product2/2
  Displ/1 -> Product4/2, Product2/1
  Constant2/1 -> Product4/1
  Gain2/1 -> Product/1

== system PTOSim_Lib/Hydraulic/Rectifying Check Valve/Valve1 ==
  DeltaP : Inport
  Av : Subsystem
  Constant : Constant  Value=PTOSimBlock.RectifyingCheckValve.rho
  Divide : Product  Inputs=/*
  Gain : Gain  Gain=PTOSimBlock.RectifyingCheckValve.k1
  Gain1 : Gain  Gain=2
  Gain2 : Gain  Gain=PTOSimBlock.RectifyingCheckValve.Cd
  Product : Product
  Product1 : Product
  Sqrt : Sqrt  SaturateOnIntegerOverflow=on
  Trigonometric Function : Trigonometry  Operator=tanh
  Qcv : Outport
  wires:
  DeltaP/1 -> Gain/1, Gain1/1, Av/1(DeltaP)
  Gain/1 -> Trigonometric Function/1
  Trigonometric Function/1 -> Product/1
  Gain1/1 -> Product/2
  Product/1 -> Divide/2
  Constant/1 -> Divide/1
  Divide/1 -> Sqrt/1
  Sqrt/1 -> Gain2/1
  Gain2/1 -> Product1/1
  Av/1(Av) -> Product1/2
  Product1/1 -> Qcv/1

== system PTOSim_Lib/Motion Conversion/Rotary to Linear Adjustable Rod/Angle Calculation for PTO ==
  angPos : Inport
  Add : Sum  Inputs=+-
  Add1 : Sum  Inputs=+-
  Constant1 : Constant  Value=PTOSimBlock.AdjustableRod.crank
  Constant2 : Constant  Value=PTOSimBlock.AdjustableRod.crank
  Constant3 : Constant  Value=PTOSimBlock.AdjustableRod.offset
  Distance btw flap joint & rod joint along x-axis : Subsystem  AncestorBlock=|
      | PTOSim_Lib/Motion Conversion/Rotary to Linear
      | Adjustable Rod/Angular to Linear
      | Velocity/Subsystem/Distance btw flap joint & rod joint
      | along x-axis
  Divide : Product  Inputs=*/
  Divide1 : Product  Inputs=*/
  Product : Product
  Product1 : Product
  Subsystem1 : Subsystem  AncestorBlock=|
      | PTOSim_Lib/Motion Conversion/Rotary to Linear
      | Adjustable Rod/Angular to Linear
      | Velocity/Subsystem
  Subsystem2 : Subsystem  AncestorBlock=|
      | PTOSim_Lib/Motion Conversion/Rotary to Linear
      | Adjustable Rod/Angular to Linear
      | Velocity/Subsystem
  Trigonometric Function : Trigonometry
  Trigonometric Function1 : Trigonometry  Operator=cos
  Cos_gamma : Outport
  Sin_gamma : Outport  Port=2
  wires:
  Trigonometric Function/1 -> Product/1
  Product/1 -> Add/1
  Distance btw flap joint & rod joint along x-axis/1(d) -> Add/2
  Constant2/1 -> Product/2
  Add/1 -> Divide/1
  Subsystem1/1(rodLength) -> Divide/2
  Divide/1 -> Cos_gamma/1
  Subsystem2/1(rodLength) -> Divide1/2
  Trigonometric Function1/1 -> Product1/1
  Constant1/1 -> Product1/2
  Product1/1 -> Add1/1
  Constant3/1 -> Add1/2
  Add1/1 -> Divide1/1
  angPos/1 -> Subsystem1/1(angPos), Subsystem2/1(angPos), Trigonometric Function1/1, Trigonometric Function/1
  Divide1/1 -> Sin_gamma/1

== system PTOSim_Lib/Motion Conversion/Rotary to Linear Adjustable Rod/Angular to Linear Position ==
  angPos : Inport
  Add1 : Sum  Inputs=+-
  Add2 : Sum  Inputs=+-
  Add5 : Sum
  Add6 : Sum  Inputs=+-
  Constant1 : Constant  Value=PTOSimBlock.AdjustableRod.rodInit
  Constant2 : Constant  Value=PTOSimBlock.AdjustableRod.crank
  Constant3 : Constant  Value=PTOSimBlock.AdjustableRod.offset
  Constant7 : Constant  Value=PTOSimBlock.AdjustableRod.crank
  Distance btw flap joint & rod joint along x-axis : Subsystem
  Math Function1 : Math  Operator=square  SignedPower=on  SaturateOnIntegerOverflow=on
  Math Function6 : Math  Operator=square  SignedPower=on  SaturateOnIntegerOverflow=on
  Product1 : Product  Inputs=**
  Product7 : Product  Inputs=**
  Sqrt2 : Sqrt  SaturateOnIntegerOverflow=on
  Trigonometric Function1 : Trigonometry  Operator=cos
  Trigonometric Function5 : Trigonometry
  linearPos : Outport
  wires:
  angPos/1 -> Trigonometric Function5/1, Trigonometric Function1/1
  Add1/1 -> linearPos/1
  Add2/1 -> Math Function1/1
  Trigonometric Function5/1 -> Product7/2
  Product7/1 -> Add6/2
  Add6/1 -> Math Function6/1
  Math Function6/1 -> Add5/2
  Add5/1 -> Sqrt2/1
  Sqrt2/1 -> Add1/2
  Constant1/1 -> Add1/1
  Constant2/1 -> Product1/1
  Trigonometric Function1/1 -> Product1/2
  Product1/1 -> Add2/1
  Constant3/1 -> Add2/2
  Math Function1/1 -> Add5/1
  Constant7/1 -> Product7/1
  Distance btw flap joint & rod joint along x-axis/1(d) -> Add6/1

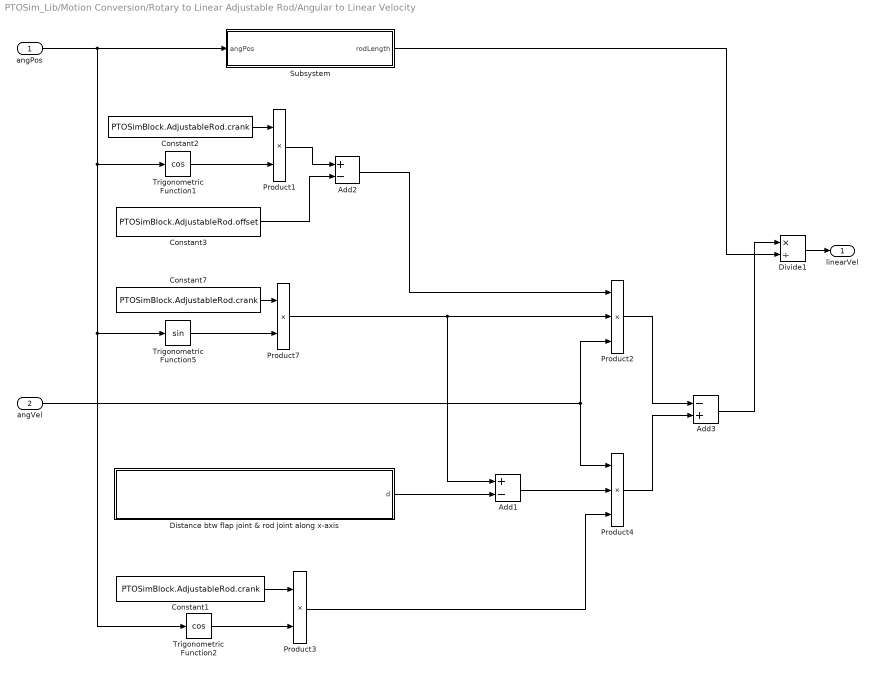
== system PTOSim_Lib/Motion Conversion/Rotary to Linear Adjustable Rod/Angular to Linear Velocity ==
  angPos : Inport
  angVel : Inport  Port=2
  Add1 : Sum  Inputs=+-
  Add2 : Sum  Inputs=+-
  Add3 : Sum  Inputs=-+
  Constant1 : Constant  Value=PTOSimBlock.AdjustableRod.crank
  Constant2 : Constant  Value=PTOSimBlock.AdjustableRod.crank
  Constant3 : Constant  Value=PTOSimBlock.AdjustableRod.offset
  Constant7 : Constant  Value=PTOSimBlock.AdjustableRod.crank
  Distance btw flap joint & rod joint along x-axis : Subsystem
  Divide1 : Product  Inputs=*/
  Product1 : Product  Inputs=**
  Product2 : Product  Inputs=***
  Product3 : Product  Inputs=**
  Product4 : Product  Inputs=***
  Product7 : Product  Inputs=**
  Subsystem : Subsystem
  Trigonometric Function1 : Trigonometry  Operator=cos
  Trigonometric Function2 : Trigonometry  Operator=cos
  Trigonometric Function5 : Trigonometry
  linearVel : Outport
  wires:
  Add2/1 -> Product2/1
  Constant2/1 -> Product1/1
  Trigonometric Function1/1 -> Product1/2
  Product1/1 -> Add2/1
  Constant3/1 -> Add2/2
  Trigonometric Function5/1 -> Product7/2
  Product7/1 -> Add1/1, Product2/2
  Constant7/1 -> Product7/1
  angVel/1 -> Product2/3, Product4/1
  Distance btw flap joint & rod joint along x-axis/1(d) -> Add1/2
  Constant1/1 -> Product3/1
  Trigonometric Function2/1 -> Product3/2
  Product3/1 -> Product4/3
  angPos/1 -> Trigonometric Function5/1, Trigonometric Function2/1, Trigonometric Function1/1, Subsystem/1(angPos)
  Add1/1 -> Product4/2
  Subsystem/1(rodLength) -> Divide1/2
  Product2/1 -> Add3/1
  Product4/1 -> Add3/2
  Add3/1 -> Divide1/1
  Divide1/1 -> linearVel/1

== system PTOSim_Lib/Motion Conversion/Rotary to Linear Crank/Angular to Linear Position ==
  angPos : Inport
  Add1 : Sum  Inputs=++-
  Add2 : Sum  Inputs=+-
  Add5 : Sum  Inputs=+-
  Constant1 : Constant  Value=PTOSimBlock.LinearCrank.rodLength
  Constant2 : Constant  Value=PTOSimBlock.LinearCrank.crank
  Constant3 : Constant  Value=PTOSimBlock.LinearCrank.offset
  Constant7 : Constant  Value=PTOSimBlock.LinearCrank.crank
  Initial Distance btw flap joint & crank joint along x-axis : Subsystem
  Math Function1 : Math  Operator=square  SignedPower=on  SaturateOnIntegerOverflow=on
  Math Function2 : Math  Operator=square  SignedPower=on  SaturateOnIntegerOverflow=on
  Product1 : Product  Inputs=**
  Product7 : Product  Inputs=**
  Sqrt2 : Sqrt  SaturateOnIntegerOverflow=on
  Trigonometric Function1 : Trigonometry  Operator=cos
  Trigonometric Function5 : Trigonometry
  linearPos : Outport
  wires:
  angPos/1 -> Trigonometric Function1/1, Trigonometric Function5/1
  Add2/1 -> Math Function1/1
  Trigonometric Function5/1 -> Product7/2
  Add5/1 -> Sqrt2/1
  Constant2/1 -> Product1/1
  Trigonometric Function1/1 -> Product1/2
  Product1/1 -> Add2/1
  Constant3/1 -> Add2/2
  Constant7/1 -> Product7/1
  Initial Distance btw flap joint & crank joint along x-axis/1(d) -> Add1/3
  Constant1/1 -> Math Function2/1
  Math Function1/1 -> Add5/2
  Sqrt2/1 -> Add1/2
  Product7/1 -> Add1/1
  Add1/1 -> linearPos/1
  Math Function2/1 -> Add5/1

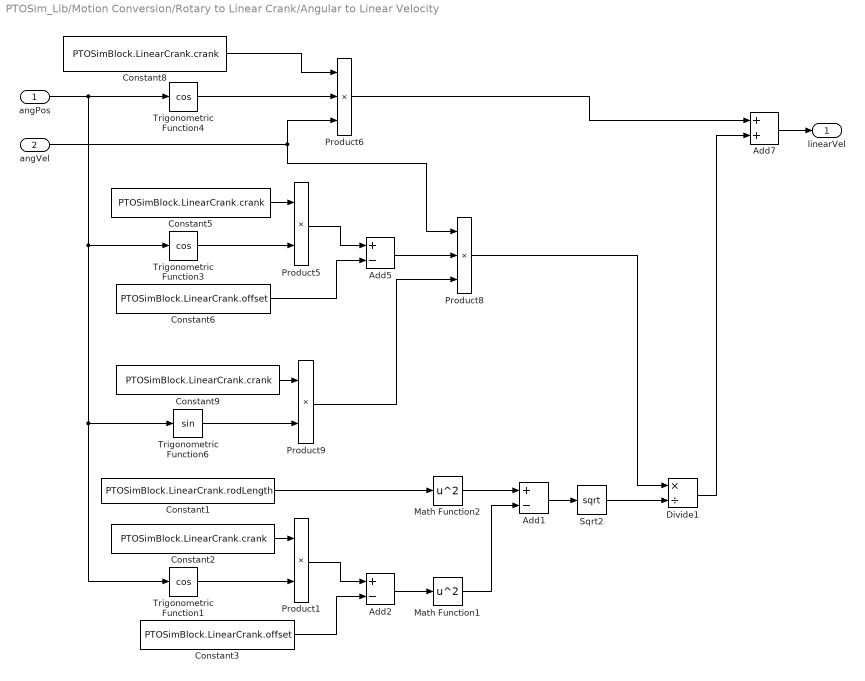
== system PTOSim_Lib/Motion Conversion/Rotary to Linear Crank/Angular to Linear Velocity ==
  angPos : Inport
  angVel : Inport  Port=2
  Add1 : Sum  Inputs=+-
  Add2 : Sum  Inputs=+-
  Add5 : Sum  Inputs=+-
  Add7 : Sum
  Constant1 : Constant  Value=PTOSimBlock.LinearCrank.rodLength
  Constant{2,5,8..9} (4 alike) : Constant  Value=PTOSimBlock.LinearCrank.crank
  Constant3 : Constant  Value=PTOSimBlock.LinearCrank.offset
  Constant6 : Constant  Value=PTOSimBlock.LinearCrank.offset
  Divide1 : Product  Inputs=*/
  Math Function1 : Math  Operator=square  SignedPower=on  SaturateOnIntegerOverflow=on
  Math Function2 : Math  Operator=square  SignedPower=on  SaturateOnIntegerOverflow=on
  Product1 : Product  Inputs=**
  Product5 : Product  Inputs=**
  Product6 : Product  Inputs=***
  Product8 : Product  Inputs=***
  Product9 : Product  Inputs=**
  Sqrt2 : Sqrt  SaturateOnIntegerOverflow=on
  Trigonometric Function1 : Trigonometry  Operator=cos
  Trigonometric Function3 : Trigonometry  Operator=cos
  Trigonometric Function4 : Trigonometry  Operator=cos
  Trigonometric Function6 : Trigonometry
  linearVel : Outport
  wires:
  Add7/1 -> linearVel/1
  Trigonometric Function4/1 -> Product6/2
  Constant8/1 -> Product6/1
  Product6/1 -> Add7/1
  Constant5/1 -> Product5/1
  Trigonometric Function3/1 -> Product5/2
  Product5/1 -> Add5/1
  Constant6/1 -> Add5/2
  Constant9/1 -> Product9/1
  Trigonometric Function6/1 -> Product9/2
  angVel/1 -> Product8/1, Product6/3
  Add5/1 -> Product8/2
  Product9/1 -> Product8/3
  angPos/1 -> Trigonometric Function1/1, Trigonometric Function6/1, Trigonometric Function3/1, Trigonometric Function4/1
  Add2/1 -> Math Function1/1
  Add1/1 -> Sqrt2/1
  Constant2/1 -> Product1/1
  Trigonometric Function1/1 -> Product1/2
  Product1/1 -> Add2/1
  Constant3/1 -> Add2/2
  Constant1/1 -> Math Function2/1
  Math Function1/1 -> Add1/2
  Sqrt2/1 -> Divide1/2
  Product8/1 -> Divide1/1
  Divide1/1 -> Add7/2
  Math Function2/1 -> Add1/1

== system PTOSim_Lib/Motion Conversion/Rotary to Linear Crank/Subsystem ==
  angle : Inport
  Add : Sum  Inputs=+-
  Add1 : Sum  Inputs=+-
  Constant : Constant
  Constant2 : Constant  Value=PTOSimBlock.LinearCrank.crank
  Constant3 : Constant  Value=PTOSimBlock.LinearCrank.offset
  Constant4 : Constant  Value=PTOSimBlock.LinearCrank.rodLength
  Divide : Product  Inputs=*/
  Product : Product
  Sqrt : Sqrt  SaturateOnIntegerOverflow=on
  Square : Math  Operator=square  SignedPower=on  SaturateOnIntegerOverflow=on
  Trigonometric Function : Trigonometry  Operator=cos
  abs(cos_gamma) : Outport
  wires:
  angle/1 -> Trigonometric Function/1
  Trigonometric Function/1 -> Product/1
  Constant2/1 -> Product/2
  Product/1 -> Add/1
  Constant3/1 -> Add/2
  Add/1 -> Divide/1
  Constant4/1 -> Divide/2
  Divide/1 -> Square/1
  Square/1 -> Add1/2
  Add1/1 -> Sqrt/1
  Constant/1 -> Add1/1
  Sqrt/1 -> abs(cos_gamma)/1

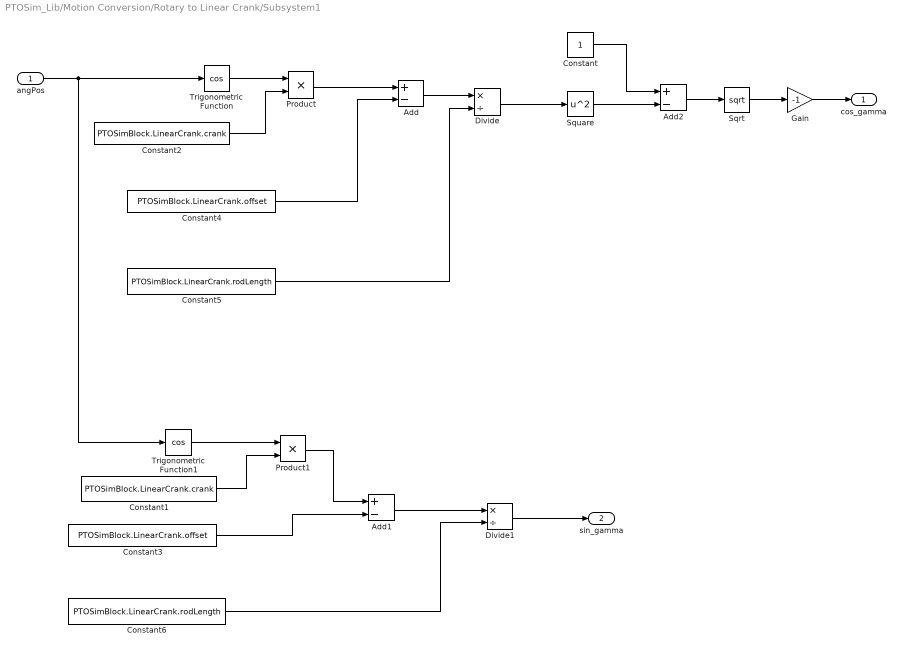
== system PTOSim_Lib/Motion Conversion/Rotary to Linear Crank/Subsystem1 ==
  angPos : Inport
  Add : Sum  Inputs=+-
  Add1 : Sum  Inputs=+-
  Add2 : Sum  Inputs=+-
  Constant : Constant
  Constant1 : Constant  Value=PTOSimBlock.LinearCrank.crank
  Constant2 : Constant  Value=PTOSimBlock.LinearCrank.crank
  Constant3 : Constant  Value=PTOSimBlock.LinearCrank.offset
  Constant4 : Constant  Value=PTOSimBlock.LinearCrank.offset
  Constant5 : Constant  Value=PTOSimBlock.LinearCrank.rodLength
  Constant6 : Constant  Value=PTOSimBlock.LinearCrank.rodLength
  Divide : Product  Inputs=*/
  Divide1 : Product  Inputs=*/
  Gain : Gain  Gain=-1
  Product : Product
  Product1 : Product
  Sqrt : Sqrt  SaturateOnIntegerOverflow=on
  Square : Math  Operator=square  SignedPower=on  SaturateOnIntegerOverflow=on
  Trigonometric Function : Trigonometry  Operator=cos
  Trigonometric Function1 : Trigonometry  Operator=cos
  cos_gamma : Outport
  sin_gamma : Outport  Port=2
  wires:
  Divide1/1 -> sin_gamma/1
  Add1/1 -> Divide1/1
  Constant3/1 -> Add1/2
  Product1/1 -> Add1/1
  Constant1/1 -> Product1/2
  Trigonometric Function1/1 -> Product1/1
  Constant6/1 -> Divide1/2
  Add/1 -> Divide/1
  Add2/1 -> Sqrt/1
  angPos/1 -> Trigonometric Function1/1, Trigonometric Function/1
  Square/1 -> Add2/2
  Product/1 -> Add/1
  Constant2/1 -> Product/2
  Trigonometric Function/1 -> Product/1
  Divide/1 -> Square/1
  Constant5/1 -> Divide/2
  Constant/1 -> Add2/1
  Constant4/1 -> Add/2
  Sqrt/1 -> Gain/1
  Gain/1 -> cos_gamma/1

== system PTOSim_Lib/Hydraulic/Hydraulic Motor/AnalyticalEfficiencyModel/FlowIdeal ==
  Displ : Inport
  ShaftSpeed : Inport  Port=2
  Constant1 : Constant  Value=PTOSimBlock.HydraulicMotorV2.Displacement
  Gain : Gain  Gain=1/((100^3)*60)
  Product : Product  Inputs=3
  FlowIdeal : Outport
  wires:
  Constant1/1 -> Product/1
  Displ/1 -> Product/2
  ShaftSpeed/1 -> Product/3
  Product/1 -> Gain/1
  Gain/1 -> FlowIdeal/1

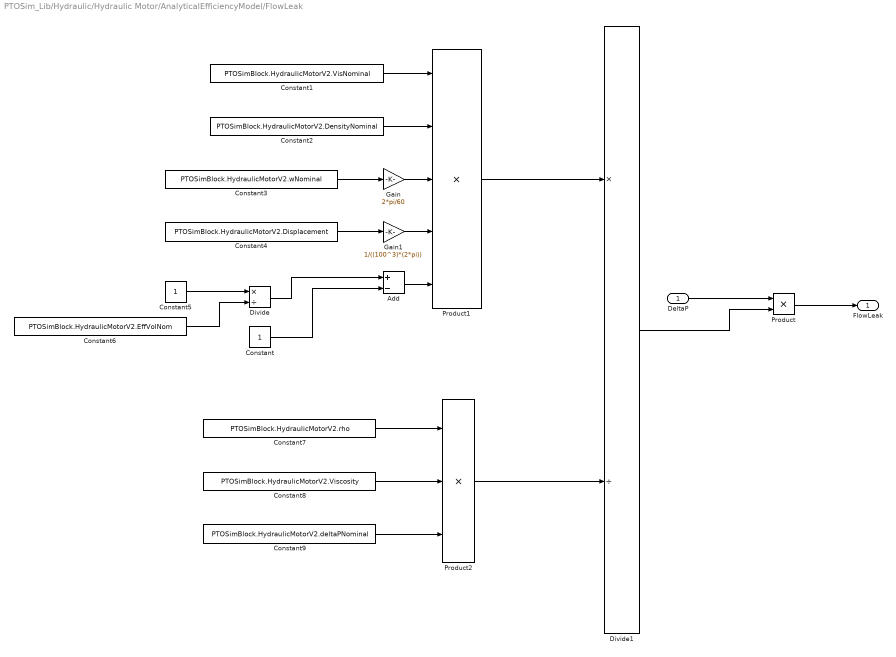
== system PTOSim_Lib/Hydraulic/Hydraulic Motor/AnalyticalEfficiencyModel/FlowLeak ==
  DeltaP : Inport
  Add : Sum  Inputs=+-
  Constant : Constant
  Constant1 : Constant  Value=PTOSimBlock.HydraulicMotorV2.VisNominal
  Constant2 : Constant  Value=PTOSimBlock.HydraulicMotorV2.DensityNominal
  Constant3 : Constant  Value=PTOSimBlock.HydraulicMotorV2.wNominal
  Constant4 : Constant  Value=PTOSimBlock.HydraulicMotorV2.Displacement
  Constant5 : Constant
  Constant6 : Constant  Value=PTOSimBlock.HydraulicMotorV2.EffVolNom
  Constant7 : Constant  Value=PTOSimBlock.HydraulicMotorV2.rho
  Constant8 : Constant  Value=PTOSimBlock.HydraulicMotorV2.Viscosity
  Constant9 : Constant  Value=PTOSimBlock.HydraulicMotorV2.deltaPNominal
  Divide : Product  Inputs=*/
  Divide1 : Product  Inputs=*/
  Gain : Gain  Gain=2*pi/60
  Gain1 : Gain  Gain=1/((100^3)*(2*pi))
  Product : Product
  Product1 : Product  Inputs=5
  Product2 : Product  Inputs=3
  FlowLeak : Outport
  wires:
  DeltaP/1 -> Product/1
  Constant1/1 -> Product1/1
  Constant2/1 -> Product1/2
  Constant3/1 -> Gain/1
  Gain/1 -> Product1/3
  Constant4/1 -> Gain1/1
  Gain1/1 -> Product1/4
  Add/1 -> Product1/5
  Constant/1 -> Add/2
  Divide/1 -> Add/1
  Constant5/1 -> Divide/1
  Constant6/1 -> Divide/2
  Product/1 -> FlowLeak/1
  Product1/1 -> Divide1/1
  Product2/1 -> Divide1/2
  Divide1/1 -> Product/2
  Constant7/1 -> Product2/1
  Constant8/1 -> Product2/2
  Constant9/1 -> Product2/3

== system PTOSim_Lib/Hydraulic/Hydraulic Motor/AnalyticalEfficiencyModel/TorqueFriction ==
  Displ : Inport
  DeltaP : Inport  Port=2
  ShaftSpeed : Inport  Port=3
  Abs : Abs
  Abs1 : Abs
  Add : Sum
  Constant : Constant  Value=PTOSimBlock.HydraulicMotorV2.TorqueNoLoad
  Constant1 : Constant  Value=PTOSimBlock.HydraulicMotorV2.TorqueVsPressure
  Constant3 : Constant  Value=PTOSimBlock.HydraulicMotorV2.wNominal
  Divide1 : Product  Inputs=*/
  Gain : Gain  Gain=4
  Gain1 : Gain  Gain=0.01
  Product : Product  Inputs=3
  Product1 : Product
  Tanh : Trigonometry  Operator=tanh
  TorqueFriccion : Outport
  wires:
  Constant/1 -> Add/1
  Product/1 -> Add/2
  Constant1/1 -> Product/1
  Displ/1 -> Abs/1
  Abs/1 -> Product/2
  DeltaP/1 -> Abs1/1
  Abs1/1 -> Product/3
  Add/1 -> Product1/2
  ShaftSpeed/1 -> Gain/1
  Constant3/1 -> Gain1/1
  Gain/1 -> Divide1/1
  Gain1/1 -> Divide1/2
  Divide1/1 -> Tanh/1
  Tanh/1 -> Product1/1
  Product1/1 -> TorqueFriccion/1

== system PTOSim_Lib/Hydraulic/Hydraulic Motor/AnalyticalEfficiencyModel/TorqueIdeal ==
  Displ : Inport
  DeltaP : Inport  Port=2
  Constant1 : Constant  Value=PTOSimBlock.HydraulicMotorV2.Displacement
  Gain : Gain  Gain=1/((100^3)*(2*pi))
  Product : Product
  Product1 : Product
  TorqueIdeal : Outport
  wires:
  Product/1 -> TorqueIdeal/1
  Gain/1 -> Product/1
  DeltaP/1 -> Product/2
  Product1/1 -> Gain/1
  Displ/1 -> Product1/2
  Constant1/1 -> Product1/1

== system PTOSim_Lib/Hydraulic/Rectifying Check Valve/Valve1/Av ==
  DeltaP : Inport
  Add : Sum
  Add1 : Sum  Inputs=+-
  Add2 : Sum  Inputs=+-
  Add3 : Sum
  Add4 : Sum
  Constant : Constant
  Constant1 : Constant  Value=PTOSimBlock.RectifyingCheckValve.Amax
  Constant2 : Constant  Value=PTOSimBlock.RectifyingCheckValve.Amin
  Constant3 : Constant  Value=PTOSimBlock.RectifyingCheckValve.pMax
  Constant4 : Constant  Value=PTOSimBlock.RectifyingCheckValve.pMin
  Constant5 : Constant  Value=PTOSimBlock.RectifyingCheckValve.Amin
  Gain : Gain  Gain=PTOSimBlock.RectifyingCheckValve.k2
  Gain1 : Gain  Gain=0.5
  Gain2 : Gain  Gain=0.5
  Product : Product
  Trigonometric Function : Trigonometry  Operator=tanh
  Av : Outport
  wires:
  Constant5/1 -> Add4/1
  Product/1 -> Add4/2
  Constant3/1 -> Add3/1
  Gain/1 -> Trigonometric Function/1
  Add2/1 -> Gain/1
  Constant/1 -> Add/2
  Add1/1 -> Gain2/1
  Constant1/1 -> Add1/1
  Trigonometric Function/1 -> Add/1
  Add3/1 -> Gain1/1
  Constant2/1 -> Add1/2
  Gain1/1 -> Add2/2
  Constant4/1 -> Add3/2
  Add/1 -> Product/1
  Gain2/1 -> Product/2
  Add4/1 -> Av/1
  DeltaP/1 -> Add2/1
